simulink model "downlink_4c2t"  (Simulink 8.7)
settings: Solver=VariableStepDiscrete  StartTime=0.0  StopTime=DUC_LINEUP_param.endTime  RelTol=1e-3
PreLoadFcn:
  | % Run the setup script when the model is opened
  | setup_downlink_4c2t;
InitFcn:
  | % Run the setup script again just before the
  | % model is run, so that any updates made
  | % after opening are applied.
  | setup_downlink_4c2t;
  | 
  | %% DSPBuilder Start
  | alt_dspbuilder_update_model(bdroot)
  | %% DSPBuilder End
values from neighbouring files (symbols this model uses):
  LUTS_DPD_CLIP =     [downlink_4c2t_dpd_clip.mat]
  PulsExtention = 128    [setup_downlink_4c2t.m]
  StartAddress1 = Iter1_Param.BaseAddr + 3200    [setup_downlink_4c2t.m]
  StartAddress2 = StartAddress1+1024    [setup_downlink_4c2t.m]
  win = [w(1:PulsExtention) ones(1,Iter0_Param.pulseLen) w(PulsExtention+1:end)]    [setup_downlink_4c2t.m]
undefined symbols (not defined in the file or in its folder): AdvDSPBChannelOutDisplay, AdvDSPBDMemDisplay, dpoly, dspba_ChannelInVis, dspba_ChannelOutVis, dspba_internal_get_channel_ports, dspba_internal_get_demux_ports, DUC_LINEUP_param, evalAionMaskParam, iq_width, Iter0_Param, latency, primtype, REG, UseDontCare, value
undefined symbols (not defined in the file): cfr0_id, cfr_Params0, cfr_Params1, clock_rate, REG_dut_id_addr
libraries: DSPBAPrim x1438, DSPBAControl x77, DSPBAModelBus x71, DSPBABase x40, downlink_4c2t_foldingcfr_3firs_lib x26, DSPBAUtilities x8, downlink_4c2t_lib x4, downlink_4c2t_cordic_lib x2, downlink_4c2t_dpd_clipper x2, DSPBAFilters x2, DSPBAWaveformSynth x2, downlink_4c2t_lduc_lib x1
(part 13 of 17)

== system downlink_4c2t/DUT/DUC_IN_PM/carrier_separation/Subsystem4 ==
  channel_in : Inport
  valid_in : Inport  Port=2
  axc0_dataout : Inport  Port=3
  axc1_dataout : Inport  Port=4
  axc2_dataout : Inport  Port=5
  axc3_dataout : Inport  Port=6
  axc4_dataout : Inport  Port=7
  axc5_dataout : Inport  Port=8
  axc6_dataout : Inport  Port=9
  axc7_dataout : Inport  Port=10
  BitExtract1 : DSPBAPrim/BitExtract  primtype=bitextract  nInputs=1  nOutputs=1  omode=Specify via dialog  otype=ufix(4)  scale=2^0  rndmethod=Unbiased  factor=1  satmethod=Symmetric  shift_vec=[0 1 2 -1]  value=1  inPortNames=[' '; ' ';]  outPortNames=[' ']  dspbaimage=dspba_prim.jpg  text=fprintf('..%d', value);  style=Optimised  visibilities=8 + 1024  version=20090407
  Const : DSPBAPrim/Const  primtype=const  nInputs=0  nOutputs=1  omode=Inherit via internal rule  otype=sfix(16)  scale=2^-15  rndmethod=Unbiased  factor=1  satmethod=Symmetric  shift_vec=[0 1 2 -1]  value=0  inPortNames=['+'; '+';]  outPortNames=[' ']  dspbaimage=dspba_prim.jpg  text=fprintf('%s', num2str(value));  style=Optimised  visibilities=8 + 1024  floatPrecision=float32_m23  version=20120820
  Const1 : DSPBAPrim/Const  primtype=const  nInputs=0  nOutputs=1  omode=Inherit via internal rule  otype=sfix(16)  scale=2^-15  rndmethod=Unbiased  factor=1  satmethod=Symmetric  shift_vec=[0 1 2 -1]  value=1  inPortNames=['+'; '+';]  outPortNames=[' ']  dspbaimage=dspba_prim.jpg  text=fprintf('%s', num2str(value));  style=Optimised  visibilities=8 + 1024  floatPrecision=float32_m23  version=20120820
  Const2 : DSPBAPrim/Const  primtype=const  nInputs=0  nOutputs=1  omode=Inherit via internal rule  otype=sfix(16)  scale=2^-15  rndmethod=Unbiased  factor=1  satmethod=Symmetric  shift_vec=[0 1 2 -1]  value=2  inPortNames=['+'; '+';]  outPortNames=[' ']  dspbaimage=dspba_prim.jpg  text=fprintf('%s', num2str(value));  style=Optimised  visibilities=8 + 1024  floatPrecision=float32_m23  version=20120820
  Const3 : DSPBAPrim/Const  primtype=const  nInputs=0  nOutputs=1  omode=Inherit via internal rule  otype=sfix(16)  scale=2^-15  rndmethod=Unbiased  factor=1  satmethod=Symmetric  shift_vec=[0 1 2 -1]  value=3  inPortNames=['+'; '+';]  outPortNames=[' ']  dspbaimage=dspba_prim.jpg  text=fprintf('%s', num2str(value));  style=Optimised  visibilities=8 + 1024  floatPrecision=float32_m23  version=20120820
  Const4 : DSPBAPrim/Const  primtype=const  nInputs=0  nOutputs=1  omode=Inherit via internal rule  otype=sfix(16)  scale=2^-15  rndmethod=Unbiased  factor=1  satmethod=Symmetric  shift_vec=[0 1 2 -1]  value=4  inPortNames=['+'; '+';]  outPortNames=[' ']  dspbaimage=dspba_prim.jpg  text=fprintf('%s', num2str(value));  style=Optimised  visibilities=8 + 1024  floatPrecision=float32_m23  version=20120820
  Const5 : DSPBAPrim/Const  primtype=const  nInputs=0  nOutputs=1  omode=Inherit via internal rule  otype=sfix(16)  scale=2^-15  rndmethod=Unbiased  factor=1  satmethod=Symmetric  shift_vec=[0 1 2 -1]  value=5  inPortNames=['+'; '+';]  outPortNames=[' ']  dspbaimage=dspba_prim.jpg  text=fprintf('%s', num2str(value));  style=Optimised  visibilities=8 + 1024  floatPrecision=float32_m23  version=20120820
  Const6 : DSPBAPrim/Const  primtype=const  nInputs=0  nOutputs=1  omode=Inherit via internal rule  otype=sfix(16)  scale=2^-15  rndmethod=Unbiased  factor=1  satmethod=Symmetric  shift_vec=[0 1 2 -1]  value=6  inPortNames=['+'; '+';]  outPortNames=[' ']  dspbaimage=dspba_prim.jpg  text=fprintf('%s', num2str(value));  style=Optimised  visibilities=8 + 1024  floatPrecision=float32_m23  version=20120820
  Const7 : DSPBAPrim/Const  primtype=const  nInputs=0  nOutputs=1  omode=Inherit via internal rule  otype=sfix(16)  scale=2^-15  rndmethod=Unbiased  factor=1  satmethod=Symmetric  shift_vec=[0 1 2 -1]  value=7  inPortNames=['+'; '+';]  outPortNames=[' ']  dspbaimage=dspba_prim.jpg  text=fprintf('%s', num2str(value));  style=Optimised  visibilities=8 + 1024  floatPrecision=float32_m23  version=20120820
  Subsystem : Subsystem
  Subsystem1 : Subsystem
  Subsystem10 : Subsystem
  Subsystem11 : Subsystem
  Subsystem12 : Subsystem
  Subsystem13 : Subsystem
  Subsystem14 : Subsystem
  Subsystem15 : Subsystem
  Subsystem2 : Subsystem
  Subsystem3 : Subsystem
  Subsystem4 : Subsystem
  Subsystem5 : Subsystem
  Subsystem6 : Subsystem
  Subsystem7 : Subsystem
  Subsystem8 : Subsystem
  Subsystem9 : Subsystem
  axc0_valid_out : Outport
  "axc0_data_out " : Outport  Port=2
  axc1_valid_out : Outport  Port=3
  axc1_data_out : Outport  Port=4
  axc2_valid_out : Outport  Port=5
  axc2_data_out : Outport  Port=6
  axc3_valid_out : Outport  Port=7
  axc3_data_out : Outport  Port=8
  axc4_valid_out : Outport  Port=9
  axc4_data_out : Outport  Port=10
  axc5_valid_out : Outport  Port=11
  axc5_data_out : Outport  Port=12
  axc6_valid_out : Outport  Port=13
  axc6_data_out : Outport  Port=14
  axc7_valid_out : Outport  Port=15
  axc7_data_out : Outport  Port=16
  wires:
  Const1/1 -> Subsystem1/2(channel_num)
  Const3/1 -> Subsystem3/2(channel_num)
  Const2/1 -> Subsystem2/2(channel_num)
  Const/1 -> Subsystem/2(channel_num)
  Subsystem/1(valid_out) -> Subsystem4/1(valid_in)
  Subsystem1/1(valid_out) -> Subsystem5/1(valid_in)
  Subsystem2/1(valid_out) -> Subsystem6/1(valid_in)
  Subsystem3/1(valid_out) -> Subsystem7/1(valid_in)
  axc0_dataout/1 -> Subsystem4/2("data_in ")
  axc1_dataout/1 -> Subsystem5/2("data_in ")
  axc2_dataout/1 -> Subsystem6/2("data_in ")
  axc3_dataout/1 -> Subsystem7/2("data_in ")
  Const4/1 -> Subsystem8/2(channel_num)
  Subsystem8/1(valid_out) -> Subsystem9/1(valid_in)
  axc4_dataout/1 -> Subsystem9/2("data_in ")
  Const6/1 -> Subsystem11/2(channel_num)
  Const5/1 -> Subsystem10/2(channel_num)
  Subsystem10/1(valid_out) -> Subsystem12/1(valid_in)
  Subsystem11/1(valid_out) -> Subsystem13/1(valid_in)
  axc5_dataout/1 -> Subsystem12/2("data_in ")
  axc6_dataout/1 -> Subsystem13/2("data_in ")
  Const7/1 -> Subsystem14/2(channel_num)
  valid_in/1 -> Subsystem10/3(valid_in), Subsystem11/3(valid_in), Subsystem14/3(valid_in), Subsystem8/3(valid_in), Subsystem3/3(valid_in), Subsystem2/3(valid_in), Subsystem1/3(valid_in), Subsystem/3(valid_in)
  channel_in/1 -> BitExtract1/1
  Subsystem14/1(valid_out) -> Subsystem15/1(valid_in)
  axc7_dataout/1 -> Subsystem15/2("data_in ")
  Subsystem4/2("data_out ") -> "axc0_data_out "/1
  Subsystem7/1(vaid_out) -> axc3_valid_out/1
  Subsystem4/1(vaid_out) -> axc0_valid_out/1
  Subsystem5/1(vaid_out) -> axc1_valid_out/1
  Subsystem5/2("data_out ") -> axc1_data_out/1
  Subsystem6/1(vaid_out) -> axc2_valid_out/1
  Subsystem6/2("data_out ") -> axc2_data_out/1
  Subsystem12/2("data_out ") -> axc5_data_out/1
  Subsystem13/1(vaid_out) -> axc6_valid_out/1
  Subsystem13/2("data_out ") -> axc6_data_out/1
  Subsystem15/1(vaid_out) -> axc7_valid_out/1
  Subsystem15/2("data_out ") -> axc7_data_out/1
  Subsystem7/2("data_out ") -> axc3_data_out/1
  Subsystem12/1(vaid_out) -> axc5_valid_out/1
  Subsystem9/2("data_out ") -> axc4_data_out/1
  Subsystem9/1(vaid_out) -> axc4_valid_out/1
  BitExtract1/1 -> Subsystem1/1(channel_in), Subsystem10/1(channel_in), Subsystem11/1(channel_in), Subsystem14/1(channel_in), Subsystem8/1(channel_in), Subsystem3/1(channel_in), Subsystem2/1(channel_in), Subsystem/1(channel_in)

== system downlink_4c2t/DUT/DUC_SUMMER_PM/Ant1_accumulator/neg_egde ==
  In1 : Inport
  And : DSPBAPrim/And  primtype=and  nInputs=2  nOutputs=1  omode=Inherit via internal rule  otype=sfix(16)  scale=2^-15  rndmethod=Unbiased  factor=1  satmethod=Symmetric  shift_vec=[0 1 2 -1]  value=0  inPortNames=[' '; ' '; ' '; ' '; ' '; ' '; ' '; ' '; ' '; ' '; ' '; ' '; ' '; ' '; ' '; ' '; ]  outPortNames=[' ']  dspbaimage=dspba_prim.jpg  text=fprintf('&');  style=Optimised  visibilities=8+2  version=20090407
  Not : DSPBAPrim/Not  primtype=not  nInputs=1  nOutputs=1  omode=Inherit via internal rule  otype=sfix(16)  scale=2^-15  rndmethod=Unbiased  factor=1  satmethod=Symmetric  shift_vec=[0 1 2 -1]  value=0  inPortNames=[' '; ' ';]  outPortNames=[' ']  dspbaimage=dspba_prim.jpg  text=fprintf('~');  style=Optimised  visibilities=8  version=20090407
  SampleDelay3 : DSPBAPrim/SampleDelay  primtype=sampdelay  nInputs=1  nOutputs=1  omode=Inherit via internal rule  otype=sfix(16)  scale=2^-15  rndmethod=Unbiased  factor=1  satmethod=Symmetric  shift_vec=[0 1 2 -1]  value=1  inPortNames=[' '; ' ';]  outPortNames=[' ']  dspbaimage=dspba_prim.jpg  text=dpoly(1, eye(1,value+1), 'z')  style=Optimised  visibilities=8 + 1024 + 2^17 + 2^18  flexible=off  slackgroup=0  augmented=0  version=20090407  advOptions=[]
  Out1 : Outport
  wires:
  In1/1 -> Not/1, SampleDelay3/1
  SampleDelay3/1 -> And/1
  Not/1 -> And/2
  And/1 -> Out1/1

== system downlink_4c2t/DUT/DUC_SUMMER_PM/Ant2_accumulator/neg_egde ==
  In1 : Inport
  And : DSPBAPrim/And  primtype=and  nInputs=2  nOutputs=1  omode=Inherit via internal rule  otype=sfix(16)  scale=2^-15  rndmethod=Unbiased  factor=1  satmethod=Symmetric  shift_vec=[0 1 2 -1]  value=0  inPortNames=[' '; ' '; ' '; ' '; ' '; ' '; ' '; ' '; ' '; ' '; ' '; ' '; ' '; ' '; ' '; ' '; ]  outPortNames=[' ']  dspbaimage=dspba_prim.jpg  text=fprintf('&');  style=Optimised  visibilities=8+2  version=20090407
  Not : DSPBAPrim/Not  primtype=not  nInputs=1  nOutputs=1  omode=Inherit via internal rule  otype=sfix(16)  scale=2^-15  rndmethod=Unbiased  factor=1  satmethod=Symmetric  shift_vec=[0 1 2 -1]  value=0  inPortNames=[' '; ' ';]  outPortNames=[' ']  dspbaimage=dspba_prim.jpg  text=fprintf('~');  style=Optimised  visibilities=8  version=20090407
  SampleDelay3 : DSPBAPrim/SampleDelay  primtype=sampdelay  nInputs=1  nOutputs=1  omode=Inherit via internal rule  otype=sfix(16)  scale=2^-15  rndmethod=Unbiased  factor=1  satmethod=Symmetric  shift_vec=[0 1 2 -1]  value=1  inPortNames=[' '; ' ';]  outPortNames=[' ']  dspbaimage=dspba_prim.jpg  text=dpoly(1, eye(1,value+1), 'z')  style=Optimised  visibilities=8 + 1024 + 2^17 + 2^18  flexible=off  slackgroup=0  augmented=0  version=20090407  advOptions=[]
  Out1 : Outport
  wires:
  In1/1 -> Not/1, SampleDelay3/1
  SampleDelay3/1 -> And/1
  Not/1 -> And/2
  And/1 -> Out1/1

== system downlink_4c2t/DUT/DUC_SUMMER_PM/carrier_separation/Subsystem4 ==
  channel_in : Inport
  valid_in : Inport  Port=2
  axc0_dataout : Inport  Port=3
  axc1_dataout : Inport  Port=4
  BitExtract1 : DSPBAPrim/BitExtract  primtype=bitextract  nInputs=1  nOutputs=1  omode=Specify via dialog  otype=ufix(2)  scale=2^0  rndmethod=Unbiased  factor=1  satmethod=Symmetric  shift_vec=[0 1 2 -1]  value=1  inPortNames=[' '; ' ';]  outPortNames=[' ']  dspbaimage=dspba_prim.jpg  text=fprintf('..%d', value);  style=Optimised  visibilities=8 + 1024  version=20090407
  Const : DSPBAPrim/Const  primtype=const  nInputs=0  nOutputs=1  omode=Inherit via internal rule  otype=sfix(16)  scale=2^-15  rndmethod=Unbiased  factor=1  satmethod=Symmetric  shift_vec=[0 1 2 -1]  value=0  inPortNames=['+'; '+';]  outPortNames=[' ']  dspbaimage=dspba_prim.jpg  text=fprintf('%s', num2str(value));  style=Optimised  visibilities=8 + 1024  floatPrecision=float32_m23  version=20120820
  Const1 : DSPBAPrim/Const  primtype=const  nInputs=0  nOutputs=1  omode=Inherit via internal rule  otype=sfix(16)  scale=2^-15  rndmethod=Unbiased  factor=1  satmethod=Symmetric  shift_vec=[0 1 2 -1]  value=1  inPortNames=['+'; '+';]  outPortNames=[' ']  dspbaimage=dspba_prim.jpg  text=fprintf('%s', num2str(value));  style=Optimised  visibilities=8 + 1024  floatPrecision=float32_m23  version=20120820
  Subsystem : Subsystem
  Subsystem1 : Subsystem
  Subsystem2 : Subsystem
  Subsystem4 : Subsystem
  axc0_valid_out : Outport
  "axc0_data_out " : Outport  Port=2
  axc1_valid_out : Outport  Port=3
  axc1_data_out : Outport  Port=4
  wires:
  BitExtract1/1 -> Subsystem/1(channel_in), Subsystem1/1(channel_in)
  Subsystem2/2("data_out ") -> axc1_data_out/1
  Subsystem2/1(vaid_out) -> axc1_valid_out/1
  Subsystem4/1(vaid_out) -> axc0_valid_out/1
  Subsystem4/2("data_out ") -> "axc0_data_out "/1
  channel_in/1 -> BitExtract1/1
  valid_in/1 -> Subsystem/3(valid_in), Subsystem1/3(valid_in)
  axc1_dataout/1 -> Subsystem2/2("data_in ")
  axc0_dataout/1 -> Subsystem4/2("data_in ")
  Subsystem1/1(valid_out) -> Subsystem2/1(valid_in)
  Subsystem/1(valid_out) -> Subsystem4/1(valid_in)
  Const/1 -> Subsystem/2(channel_num)
  Const1/1 -> Subsystem1/2(channel_num)

== system downlink_4c2t/DUT/LDUC/Mixer_Summer/COMPLEX_MIXER ==
  a : Inport
  v : Inport  Port=2
  c : Inport  Port=3
  sync_pulse : Inport  Port=4
  ComplexMixer : DSPBAWaveformSynth/ComplexMixer  nInputRate=DUC_LINEUP_param.CM.SampleRate  nchan=DUC_LINEUP_param.CM.No_Of_Complex_chan  nfreq=DUC_LINEUP_param.CM.No_Of_Complex_Freq  latency=4  version=20090407
  Const1 : DSPBAPrim/Const  primtype=const  nInputs=0  nOutputs=1  omode=Specify via dialog  otype=ufix(24)  scale=2^-0  rndmethod=Unbiased  factor=1  satmethod=Symmetric  shift_vec=[0 1 2 -1]  value=[0 0]  inPortNames=['+'; '+';]  outPortNames=[' ']  dspbaimage=dspba_prim.jpg  text=fprintf('%s', num2str(value));  style=Optimised  visibilities=8 + 1024  floatPrecision=float32_m23  version=20120820
  Const25 : DSPBAPrim/Const  primtype=const  nInputs=0  nOutputs=1  omode=Inherit via internal rule  otype=sfix(16)  scale=2^-15  rndmethod=Unbiased  factor=1  satmethod=Symmetric  shift_vec=[0 1 2 -1]  value=0  inPortNames=['+'; '+';]  outPortNames=[' ']  dspbaimage=dspba_prim.jpg  text=fprintf('%s', num2str(value));  style=Optimised  visibilities=8 + 1024  floatPrecision=float32_m23  version=20120820
  Delay Module : Subsystem
  Demux : Demux  Outputs=2
  IQ_Splitter : Subsystem
  Mux : Mux  Inputs=2
  Mux1 : Mux  Inputs=2
  NCO1 : DSPBAWaveformSynth/NCO  outputRate=DUC_LINEUP_param.NCO.SampleRate  otype=sfix(DUC_LINEUP_param.NCO.Data_type)  scale=2^-DUC_LINEUP_param.NCO.scaling_value  expSFDR=96.32  accumBitWidth=DUC_LINEUP_param.NCO.Acumulater_bit_wid  accumPrecision=+/- 3.6621  phaseIncrAndInv=DUC_LINEUP_param.A12xC_NCO.Freq_word  phaseIncrInMHz="[0  0  0  0  0  0  0  0]"  phaseIncrAndInvMap=DUC_LINEUP_param.A12xC_NCO.base_addr  rwmode=Read/Write  exposebus=off  outWidth=2  tableSize=8  latency=19  version=20090407
  Terminator28 : Terminator
  Terminator8 : Terminator
  Terminator9 : Terminator
  scale1_ComplexMixer : DSPBABase/Scale  otype=sfix(DUC_LINEUP_param.output_word_length)  scale=2^-DUC_LINEUP_param.output_fraction_length  rndmethod=Truncate  factor=[1 1]  satmethod=Symmetric  shift_vec=[0 0]  latency=6  wideSimulation=off  version=20090407
  out_I : Outport
  out_q : Outport  Port=2
  q_v : Outport  Port=3
  q_c : Outport  Port=4
  wires:
  Delay Module/4(Out_Chan) -> Terminator9/1
  v/1 -> IQ_Splitter/2(valid)
  NCO1/1 -> ComplexMixer/5
  Delay Module/3(Out_Valid) -> Terminator8/1
  ComplexMixer/1 -> Mux/1
  scale1_ComplexMixer/3 -> q_c/1
  scale1_ComplexMixer/4 -> Terminator28/1
  Mux/1 -> scale1_ComplexMixer/1
  IQ_Splitter/4(Out_channel) -> Delay Module/4(In_Chann), NCO1/1
  scale1_ComplexMixer/2 -> q_v/1
  c/1 -> IQ_Splitter/3(channel)
  ComplexMixer/2 -> Mux/2
  IQ_Splitter/1(Out_data_I) -> Delay Module/1(In_Data1)
  ComplexMixer/3 -> scale1_ComplexMixer/2
  a/1 -> IQ_Splitter/1(data)
  Delay Module/1(Out_Data1) -> ComplexMixer/1
  NCO1/3 -> ComplexMixer/3
  ComplexMixer/4 -> scale1_ComplexMixer/3
  NCO1/4 -> ComplexMixer/4
  NCO1/2 -> ComplexMixer/6
  Const1/1 -> NCO1/3
  Const25/1 -> scale1_ComplexMixer/4
  scale1_ComplexMixer/1 -> Demux/1
  Demux/1 -> out_I/1
  Demux/2 -> out_q/1
  IQ_Splitter/2(Out_data_Q) -> Delay Module/2(In_Data2)
  IQ_Splitter/3(Out_valid) -> NCO1/2, Delay Module/3(In_Valid)
  Mux1/1 -> NCO1/4
  sync_pulse/1 -> Mux1/2, Mux1/1
  Delay Module/2(Out_Data2) -> ComplexMixer/2

== system downlink_4c2t/DUT/LDUC/Mixer_Summer/SUMMER ==
  a : Inport
  a1 : Inport  Port=2
  v : Inport  Port=3
  c : Inport  Port=4
  sum_shift : Inport  Port=5
  IQ_Summer : Subsystem
  Terminator7 : Terminator
  scale_HB_filter5 : DSPBABase/Scale  otype=sfix(DUC_LINEUP_param.output_word_length)  scale=2^-DUC_LINEUP_param.output_fraction_length  rndmethod=Truncate  factor=1  satmethod=Symmetric  shift_vec=[0 -1 -2 -2]  latency=6  wideSimulation=off  version=20090407
  q : Outport
  q_v : Outport  Port=2
  q_c : Outport  Port=3
  wires:
  v/1 -> IQ_Summer/3(valid)
  c/1 -> IQ_Summer/4(chann)
  scale_HB_filter5/2 -> q_v/1
  scale_HB_filter5/3 -> q_c/1
  scale_HB_filter5/4 -> Terminator7/1
  IQ_Summer/2(out_valid) -> scale_HB_filter5/2
  a/1 -> IQ_Summer/1(data0)
  scale_HB_filter5/1 -> q/1
  IQ_Summer/1(Out_data) -> scale_HB_filter5/1
  IQ_Summer/3(Out_chann) -> scale_HB_filter5/3
  a1/1 -> IQ_Summer/2(data1)
  sum_shift/1 -> scale_HB_filter5/4

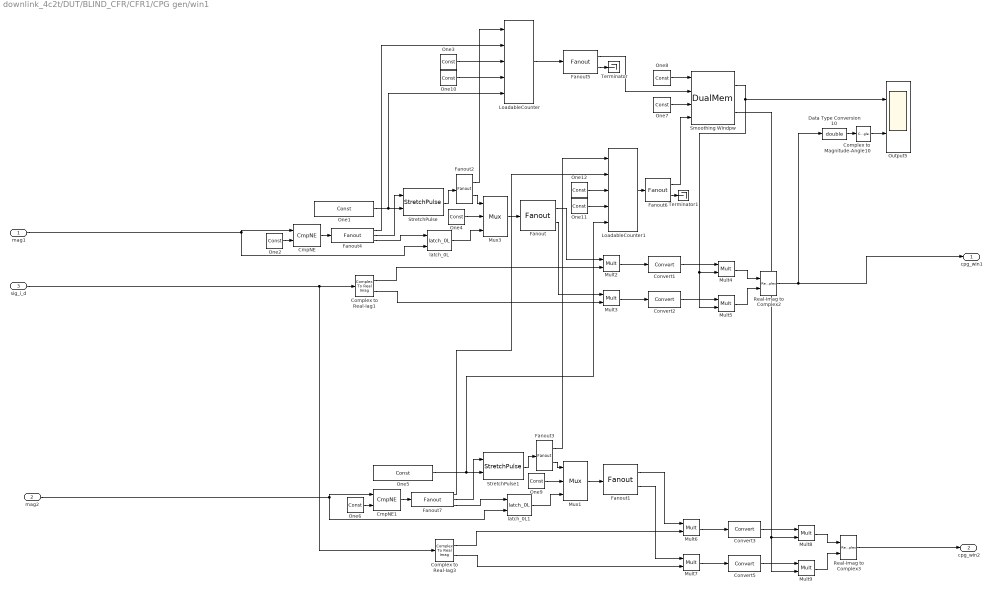
== system downlink_4c2t/DUT/BLIND_CFR/CFR1/CPG gen/win1 ==
  mag1 : Inport
  mag2 : Inport  Port=2
  sig_i_d : Inport  Port=3
  CmpNE : DSPBAPrim/CmpNE  primtype=cmpne  nInputs=2  nOutputs=1  omode=boolean  otype=sfix(16)  scale=2^-15  rndmethod=Unbiased  factor=1  satmethod=Symmetric  shift_vec=[0 1 2 -1]  value=0  inPortNames=[' '; ' ';]  outPortNames=[' ']  dspbaimage=dspba_prim.jpg  text=fprintf('~=');  style=Optimised  visibilities=0  advOptions=[]  version=20130117
  CmpNE1 : DSPBAPrim/CmpNE  primtype=cmpne  nInputs=2  nOutputs=1  omode=boolean  otype=sfix(16)  scale=2^-15  rndmethod=Unbiased  factor=1  satmethod=Symmetric  shift_vec=[0 1 2 -1]  value=0  inPortNames=[' '; ' ';]  outPortNames=[' ']  dspbaimage=dspba_prim.jpg  text=fprintf('~=');  style=Optimised  visibilities=0  advOptions=[]  version=20130117
  Complex to Magnitude-Angle10 : ComplexToMagnitudeAngle  Output=Magnitude
  Complex to Real-Iag1 : ComplexToRealImag
  Complex to Real-Iag3 : ComplexToRealImag
  Convert{1..3,5} (4 alike) : DSPBAPrim/Convert  primtype=convert  nInputs=1  nOutputs=1  omode=Specify via dialog  otype=sfix(16)  scale=2^-(15)  rndmethod=Unbiased  factor=1  satmethod=None  shift_vec=[0 1 2 -1]  value=round([0:255]/17)  inPortNames=[' '; ' ';]  outPortNames=[' '; 'c']  dspbaimage=dspba_prim.jpg  text=fprintf('convert');  style=Optimised  visibilities=8+64+256  clipdetect=off  floatPrecision=float32_m23  advOptions=[]  version=20130211
  Data Type Conversion10 : DataTypeConversion  OutDataTypeStr=double
  Fanout{,1..3,5..6} (6 alike) : DSPBAPrim/Fanout  primtype=fanout  nInputs=1  nOutputs=evalAionMaskParam(gcb,'value',1)  omode=Inherit via internal rule  otype=sfix(16)  scale=2^-15  rndmethod=Unbiased  factor=1  satmethod=Symmetric  shift_vec=[0 1 2 -1]  value=2  inPortNames=[' '; ' ';]  outPortNames=[' ']  dspbaimage=dspba_prim.jpg  text=fprintf('fanout')  style=Optimised  visibilities=2^10+2^18  version=20150501  uninit=off
  Fanout4 : DSPBAPrim/Fanout  primtype=fanout  nInputs=1  nOutputs=evalAionMaskParam(gcb,'value',1)  omode=Inherit via internal rule  otype=sfix(16)  scale=2^-15  rndmethod=Unbiased  factor=1  satmethod=Symmetric  shift_vec=[0 1 2 -1]  value=3  inPortNames=[' '; ' ';]  outPortNames=[' ']  dspbaimage=dspba_prim.jpg  text=fprintf('fanout')  style=Optimised  visibilities=2^10+2^18  version=20150501  uninit=off
  Fanout7 : DSPBAPrim/Fanout  primtype=fanout  nInputs=1  nOutputs=evalAionMaskParam(gcb,'value',1)  omode=Inherit via internal rule  otype=sfix(16)  scale=2^-15  rndmethod=Unbiased  factor=1  satmethod=Symmetric  shift_vec=[0 1 2 -1]  value=3  inPortNames=[' '; ' ';]  outPortNames=[' ']  dspbaimage=dspba_prim.jpg  text=fprintf('fanout')  style=Optimised  visibilities=2^10+2^18  version=20150501  uninit=off
  LoadableCounter : DSPBAPrim/LoadableCounter  primtype=loadablecounter  nInputs=5  nOutputs=1  omode=Inherit via internal rule  otype=ufix(16)  scale=2^-0  rndmethod=Unbiased  factor=1  satmethod=Symmetric  shift_vec=[0 1 2 -1]  value=[0 length(win) 1]  inPortNames=['en';'ld';'i ';'s ';'m ']  outPortNames=[' ']  dspbaimage=dspba_prim.jpg  text=fprintf('loadable\ncounter\n[%d %d %d]', value(1), value(2), value(3));  style=Optimised  visibilities=8 + 1024  version=20090407
  LoadableCounter1 : DSPBAPrim/LoadableCounter  primtype=loadablecounter  nInputs=5  nOutputs=1  omode=Inherit via internal rule  otype=ufix(16)  scale=2^-0  rndmethod=Unbiased  factor=1  satmethod=Symmetric  shift_vec=[0 1 2 -1]  value=[0 length(win) 1]  inPortNames=['en';'ld';'i ';'s ';'m ']  outPortNames=[' ']  dspbaimage=dspba_prim.jpg  text=fprintf('loadable\ncounter\n[%d %d %d]', value(1), value(2), value(3));  style=Optimised  visibilities=8 + 1024  version=20090407
  Mult{2..9} (8 alike) : DSPBAPrim/Mult  primtype=mult  nInputs=2  nOutputs=1  omode=Inherit via internal rule  otype=sfix(16)  scale=2^-15  rndmethod=Unbiased  factor=1  satmethod=Symmetric  shift_vec=[0 1 2 -1]  value=0  inPortNames=[' '; ' ';]  outPortNames=[' ']  dspbaimage=dspba_prim.jpg  text=fprintf('X');  style=Optimised  visibilities=8+2^18+2^19  floatPrecision=float32_m23  floatRounding=correct  advOptions=[]  version=20130115
  Mux1 : DSPBAPrim/Mux  primtype=mux  nInputs=evalAionMaskParam(gcb,'value',1)+1  nOutputs=1  omode=Inherit via internal rule  otype=sfix(16)  scale=2^-15  rndmethod=Unbiased  factor=1  satmethod=Symmetric  shift_vec=[0 1 2 -1]  value=2  inPortNames=['s'; 'd0'; 'd1'; 'd2'; 'd3'; 'd4'; 'd5'; 'd6'; 'd7'; 'd8'; 'd9';]  outPortNames=[' ']  dspbaimage=dspba_prim.jpg  text=fprintf('%s', primtype);  style=Optimised  visibilities=1032  version=20131025
  Mux3 : DSPBAPrim/Mux  primtype=mux  nInputs=evalAionMaskParam(gcb,'value',1)+1  nOutputs=1  omode=Inherit via internal rule  otype=sfix(16)  scale=2^-15  rndmethod=Unbiased  factor=1  satmethod=Symmetric  shift_vec=[0 1 2 -1]  value=2  inPortNames=['s'; 'd0'; 'd1'; 'd2'; 'd3'; 'd4'; 'd5'; 'd6'; 'd7'; 'd8'; 'd9';]  outPortNames=[' ']  dspbaimage=dspba_prim.jpg  text=fprintf('%s', primtype);  style=Optimised  visibilities=1032  version=20131025
  One1 : DSPBAPrim/Const  primtype=const  nInputs=0  nOutputs=1  omode=Specify via dialog  otype=uint(10)  scale=2^0  rndmethod=Unbiased  factor=1  satmethod=Symmetric  shift_vec=[0 1 2 -1]  value=Iter0_Param.winLen  inPortNames=['+'; '+';]  outPortNames=[' ']  dspbaimage=dspba_prim.jpg  text=fprintf('%s', num2str(value));  style=Optimised  visibilities=8 + 1024  floatPrecision=float32_m23  version=20120820
  One10 : DSPBAPrim/Const  primtype=const  nInputs=0  nOutputs=1  omode=Specify via dialog  otype=uint(10)  scale=2^0  rndmethod=Unbiased  factor=1  satmethod=Symmetric  shift_vec=[0 1 2 -1]  value=1  inPortNames=['+'; '+';]  outPortNames=[' ']  dspbaimage=dspba_prim.jpg  text=fprintf('%s', num2str(value));  style=Optimised  visibilities=8 + 1024  floatPrecision=float32_m23  version=20120820
  One11 : DSPBAPrim/Const  primtype=const  nInputs=0  nOutputs=1  omode=Specify via dialog  otype=uint(10)  scale=2^0  rndmethod=Unbiased  factor=1  satmethod=Symmetric  shift_vec=[0 1 2 -1]  value=1  inPortNames=['+'; '+';]  outPortNames=[' ']  dspbaimage=dspba_prim.jpg  text=fprintf('%s', num2str(value));  style=Optimised  visibilities=8 + 1024  floatPrecision=float32_m23  version=20120820
  One12 : DSPBAPrim/Const  primtype=const  nInputs=0  nOutputs=1  omode=Specify via dialog  otype=uint(10)  scale=2^0  rndmethod=Unbiased  factor=1  satmethod=Symmetric  shift_vec=[0 1 2 -1]  value=0  inPortNames=['+'; '+';]  outPortNames=[' ']  dspbaimage=dspba_prim.jpg  text=fprintf('%s', num2str(value));  style=Optimised  visibilities=8 + 1024  floatPrecision=float32_m23  version=20120820
  One2 : DSPBAPrim/Const  primtype=const  nInputs=0  nOutputs=1  omode=Inherit via internal rule  otype=sfix(16)  scale=2^-15  rndmethod=Unbiased  factor=1  satmethod=Symmetric  shift_vec=[0 1 2 -1]  value=0  inPortNames=['+'; '+';]  outPortNames=[' ']  dspbaimage=dspba_prim.jpg  text=fprintf('%s', num2str(value));  style=Optimised  visibilities=8 + 1024  floatPrecision=float32_m23  version=20120820
  One3 : DSPBAPrim/Const  primtype=const  nInputs=0  nOutputs=1  omode=Specify via dialog  otype=uint(10)  scale=2^0  rndmethod=Unbiased  factor=1  satmethod=Symmetric  shift_vec=[0 1 2 -1]  value=0  inPortNames=['+'; '+';]  outPortNames=[' ']  dspbaimage=dspba_prim.jpg  text=fprintf('%s', num2str(value));  style=Optimised  visibilities=8 + 1024  floatPrecision=float32_m23  version=20120820
  One4 : DSPBAPrim/Const  primtype=const  nInputs=0  nOutputs=1  omode=Specify via dialog  otype=ufix(16)  scale=2^-15  rndmethod=Unbiased  factor=1  satmethod=Symmetric  shift_vec=[0 1 2 -1]  value=0  inPortNames=['+'; '+';]  outPortNames=[' ']  dspbaimage=dspba_prim.jpg  text=fprintf('%s', num2str(value));  style=Optimised  visibilities=8 + 1024  floatPrecision=float32_m23  version=20120820
  One5 : DSPBAPrim/Const  primtype=const  nInputs=0  nOutputs=1  omode=Specify via dialog  otype=uint(10)  scale=2^0  rndmethod=Unbiased  factor=1  satmethod=Symmetric  shift_vec=[0 1 2 -1]  value=Iter0_Param.winLen  inPortNames=['+'; '+';]  outPortNames=[' ']  dspbaimage=dspba_prim.jpg  text=fprintf('%s', num2str(value));  style=Optimised  visibilities=8 + 1024  floatPrecision=float32_m23  version=20120820
  One6 : DSPBAPrim/Const  primtype=const  nInputs=0  nOutputs=1  omode=Inherit via internal rule  otype=sfix(16)  scale=2^-15  rndmethod=Unbiased  factor=1  satmethod=Symmetric  shift_vec=[0 1 2 -1]  value=0  inPortNames=['+'; '+';]  outPortNames=[' ']  dspbaimage=dspba_prim.jpg  text=fprintf('%s', num2str(value));  style=Optimised  visibilities=8 + 1024  floatPrecision=float32_m23  version=20120820
  One7 : DSPBAPrim/Const  primtype=const  nInputs=0  nOutputs=1  omode=boolean  otype=sfix(16)  scale=2^-15  rndmethod=Unbiased  factor=1  satmethod=Symmetric  shift_vec=[0 1 2 -1]  value=0  inPortNames=['+'; '+';]  outPortNames=[' ']  dspbaimage=dspba_prim.jpg  text=fprintf('%s', num2str(value));  style=Optimised  visibilities=8 + 1024  floatPrecision=float32_m23  version=20120820
  One8 : DSPBAPrim/Const  primtype=const  nInputs=0  nOutputs=1  omode=Specify via dialog  otype=sfix(16)  scale=2^-15  rndmethod=Unbiased  factor=1  satmethod=Symmetric  shift_vec=[0 1 2 -1]  value=0  inPortNames=['+'; '+';]  outPortNames=[' ']  dspbaimage=dspba_prim.jpg  text=fprintf('%s', num2str(value));  style=Optimised  visibilities=8 + 1024  floatPrecision=float32_m23  version=20120820
  One9 : DSPBAPrim/Const  primtype=const  nInputs=0  nOutputs=1  omode=Specify via dialog  otype=ufix(16)  scale=2^-15  rndmethod=Unbiased  factor=1  satmethod=Symmetric  shift_vec=[0 1 2 -1]  value=0  inPortNames=['+'; '+';]  outPortNames=[' ']  dspbaimage=dspba_prim.jpg  text=fprintf('%s', num2str(value));  style=Optimised  visibilities=8 + 1024  floatPrecision=float32_m23  version=20120820
  Output5 : Scope  NumInputPorts=2
  Real-Imag to Complex2 : RealImagToComplex
  Real-Imag to Complex3 : RealImagToComplex
  Smoothing Windpw : DSPBAPrim/DualMem  primtype=dualmem  nInputs=4  nOutputs=2  omode=Inherit via internal rule  otype=sfix(16)  scale=2^-15  rndmethod=Unbiased  factor=1  satmethod=Symmetric  shift_vec=[0 1 2 -1]  value=fi(win,1,16,15)  inPortNames=['d1'; 'a1'; 'w1'; 'a2']  outPortNames=['q1'; 'q2']  dspbaimage=dspba_prim.jpg  text=fprintf('dmem%s',AdvDSPBDMemDisplay(UseDontCare));  style=Optimised  visibilities=8 + 1024 + 2^17  UseDontCare=on  TwinWritePorts=off  version=20141001
  StretchPulse : DSPBAControl/StretchPulse
  StretchPulse1 : DSPBAControl/StretchPulse
  Terminator : Terminator
  Terminator1 : Terminator
  latch_0L : DSPBAControl/latch_0L
  latch_0L1 : DSPBAControl/latch_0L
  cpg_win1 : Outport
  cpg_win2 : Outport  Port=2
  wires:
  Fanout1/2 -> Mult7/1
  Fanout1/1 -> Mult6/1
  Mux1/1 -> Fanout1/1
  Fanout/2 -> Mult3/1
  Fanout/1 -> Mult2/1
  Mux3/1 -> Fanout/1
  LoadableCounter1/1 -> Fanout6/1
  One11/1 -> LoadableCounter1/4
  One12/1 -> LoadableCounter1/3
  One10/1 -> LoadableCounter/4
  One3/1 -> LoadableCounter/3
  Complex to Magnitude-Angle10/1 -> Output5/2
  Data Type Conversion10/1 -> Complex to Magnitude-Angle10/1
  latch_0L/1 -> Mux3/3
  One4/1 -> Mux3/2
  One2/1 -> CmpNE/2
  Convert1/1 -> Mult4/1
  Mult4/1 -> Real-Imag to Complex2/1
  Mult5/1 -> Real-Imag to Complex2/2
  Convert2/1 -> Mult5/1
  Real-Imag to Complex2/1 -> cpg_win1/1, Data Type Conversion10/1
  Smoothing Windpw/1 -> Output5/1, Mult4/2, Mult5/2
  One1/1 -> StretchPulse/2, LoadableCounter/5
  latch_0L1/1 -> Mux1/3
  One9/1 -> Mux1/2
  Smoothing Windpw/2 -> Mult8/2, Mult9/2
  Convert5/1 -> Mult9/1
  Mult6/1 -> Convert3/1
  Convert3/1 -> Mult8/1
  sig_i_d/1 -> Complex to Real-Iag1/1, Complex to Real-Iag3/1
  Mult8/1 -> Real-Imag to Complex3/1
  mag2/1 -> latch_0L1/2, CmpNE1/1
  Mult7/1 -> Convert5/1
  Mult9/1 -> Real-Imag to Complex3/2
  Complex to Real-Iag3/2 -> Mult7/2
  One5/1 -> StretchPulse1/2, LoadableCounter1/5
  One6/1 -> CmpNE1/2
  Complex to Real-Iag3/1 -> Mult6/2
  Complex to Real-Iag1/1 -> Mult2/2
  Mult2/1 -> Convert1/1
  Mult3/1 -> Convert2/1
  Complex to Real-Iag1/2 -> Mult3/2
  Real-Imag to Complex3/1 -> cpg_win2/1
  One7/1 -> Smoothing Windpw/3
  One8/1 -> Smoothing Windpw/1
  mag1/1 -> CmpNE/1, latch_0L/2
  Fanout2/2 -> Mux3/1
  StretchPulse/1 -> Fanout2/1
  Fanout2/1 -> LoadableCounter/1
  Fanout3/2 -> Mux1/1
  StretchPulse1/1 -> Fanout3/1
  Fanout3/1 -> LoadableCounter1/1
  LoadableCounter/1 -> Fanout5/1
  Fanout5/1 -> Smoothing Windpw/2
  Fanout6/1 -> Smoothing Windpw/4
  Fanout5/2 -> Terminator/1
  Fanout6/2 -> Terminator1/1
  CmpNE/1 -> Fanout4/1
  Fanout4/3 -> latch_0L/1
  Fanout4/2 -> StretchPulse/1
  Fanout4/1 -> LoadableCounter/2
  CmpNE1/1 -> Fanout7/1
  Fanout7/3 -> latch_0L1/1
  Fanout7/2 -> StretchPulse1/1
  Fanout7/1 -> LoadableCounter1/2

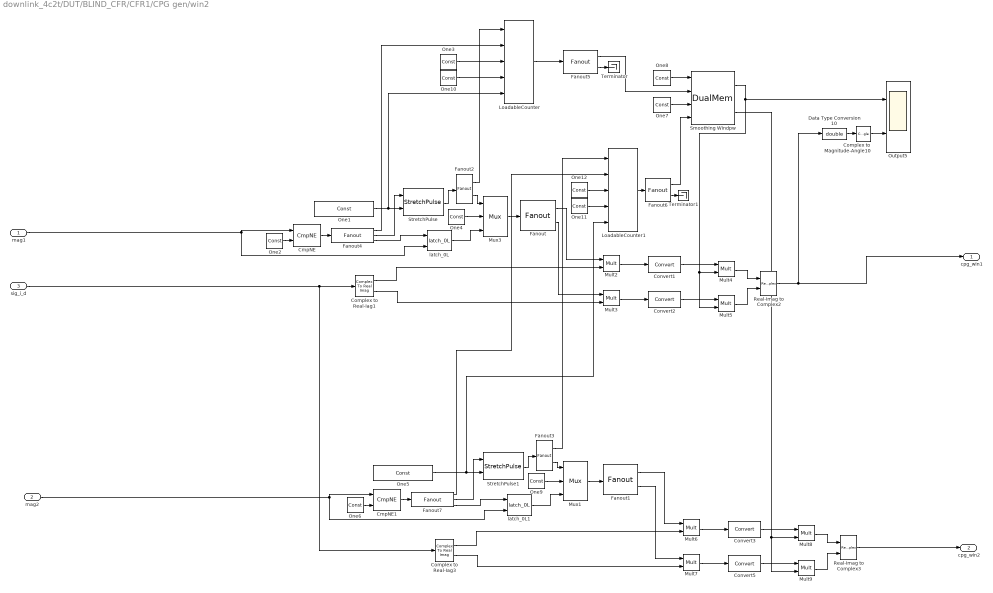
== system downlink_4c2t/DUT/BLIND_CFR/CFR1/CPG gen/win2 ==
  mag1 : Inport
  mag2 : Inport  Port=2
  sig_i_d : Inport  Port=3
  CmpNE : DSPBAPrim/CmpNE  primtype=cmpne  nInputs=2  nOutputs=1  omode=boolean  otype=sfix(16)  scale=2^-15  rndmethod=Unbiased  factor=1  satmethod=Symmetric  shift_vec=[0 1 2 -1]  value=0  inPortNames=[' '; ' ';]  outPortNames=[' ']  dspbaimage=dspba_prim.jpg  text=fprintf('~=');  style=Optimised  visibilities=0  advOptions=[]  version=20130117
  CmpNE1 : DSPBAPrim/CmpNE  primtype=cmpne  nInputs=2  nOutputs=1  omode=boolean  otype=sfix(16)  scale=2^-15  rndmethod=Unbiased  factor=1  satmethod=Symmetric  shift_vec=[0 1 2 -1]  value=0  inPortNames=[' '; ' ';]  outPortNames=[' ']  dspbaimage=dspba_prim.jpg  text=fprintf('~=');  style=Optimised  visibilities=0  advOptions=[]  version=20130117
  Complex to Magnitude-Angle10 : ComplexToMagnitudeAngle  Output=Magnitude
  Complex to Real-Iag1 : ComplexToRealImag
  Complex to Real-Iag3 : ComplexToRealImag
  Convert{1..3,5} (4 alike) : DSPBAPrim/Convert  primtype=convert  nInputs=1  nOutputs=1  omode=Specify via dialog  otype=sfix(16)  scale=2^-(15)  rndmethod=Unbiased  factor=1  satmethod=None  shift_vec=[0 1 2 -1]  value=round([0:255]/17)  inPortNames=[' '; ' ';]  outPortNames=[' '; 'c']  dspbaimage=dspba_prim.jpg  text=fprintf('convert');  style=Optimised  visibilities=8+64+256  clipdetect=off  floatPrecision=float32_m23  advOptions=[]  version=20130211
  Data Type Conversion10 : DataTypeConversion  OutDataTypeStr=double
  Fanout{,1..3,5..6} (6 alike) : DSPBAPrim/Fanout  primtype=fanout  nInputs=1  nOutputs=evalAionMaskParam(gcb,'value',1)  omode=Inherit via internal rule  otype=sfix(16)  scale=2^-15  rndmethod=Unbiased  factor=1  satmethod=Symmetric  shift_vec=[0 1 2 -1]  value=2  inPortNames=[' '; ' ';]  outPortNames=[' ']  dspbaimage=dspba_prim.jpg  text=fprintf('fanout')  style=Optimised  visibilities=2^10+2^18  version=20150501  uninit=off
  Fanout4 : DSPBAPrim/Fanout  primtype=fanout  nInputs=1  nOutputs=evalAionMaskParam(gcb,'value',1)  omode=Inherit via internal rule  otype=sfix(16)  scale=2^-15  rndmethod=Unbiased  factor=1  satmethod=Symmetric  shift_vec=[0 1 2 -1]  value=3  inPortNames=[' '; ' ';]  outPortNames=[' ']  dspbaimage=dspba_prim.jpg  text=fprintf('fanout')  style=Optimised  visibilities=2^10+2^18  version=20150501  uninit=off
  Fanout7 : DSPBAPrim/Fanout  primtype=fanout  nInputs=1  nOutputs=evalAionMaskParam(gcb,'value',1)  omode=Inherit via internal rule  otype=sfix(16)  scale=2^-15  rndmethod=Unbiased  factor=1  satmethod=Symmetric  shift_vec=[0 1 2 -1]  value=3  inPortNames=[' '; ' ';]  outPortNames=[' ']  dspbaimage=dspba_prim.jpg  text=fprintf('fanout')  style=Optimised  visibilities=2^10+2^18  version=20150501  uninit=off
  LoadableCounter : DSPBAPrim/LoadableCounter  primtype=loadablecounter  nInputs=5  nOutputs=1  omode=Inherit via internal rule  otype=ufix(16)  scale=2^-0  rndmethod=Unbiased  factor=1  satmethod=Symmetric  shift_vec=[0 1 2 -1]  value=[0 length(win) 1]  inPortNames=['en';'ld';'i ';'s ';'m ']  outPortNames=[' ']  dspbaimage=dspba_prim.jpg  text=fprintf('loadable\ncounter\n[%d %d %d]', value(1), value(2), value(3));  style=Optimised  visibilities=8 + 1024  version=20090407
  LoadableCounter1 : DSPBAPrim/LoadableCounter  primtype=loadablecounter  nInputs=5  nOutputs=1  omode=Inherit via internal rule  otype=ufix(16)  scale=2^-0  rndmethod=Unbiased  factor=1  satmethod=Symmetric  shift_vec=[0 1 2 -1]  value=[0 length(win) 1]  inPortNames=['en';'ld';'i ';'s ';'m ']  outPortNames=[' ']  dspbaimage=dspba_prim.jpg  text=fprintf('loadable\ncounter\n[%d %d %d]', value(1), value(2), value(3));  style=Optimised  visibilities=8 + 1024  version=20090407
  Mult{2..9} (8 alike) : DSPBAPrim/Mult  primtype=mult  nInputs=2  nOutputs=1  omode=Inherit via internal rule  otype=sfix(16)  scale=2^-15  rndmethod=Unbiased  factor=1  satmethod=Symmetric  shift_vec=[0 1 2 -1]  value=0  inPortNames=[' '; ' ';]  outPortNames=[' ']  dspbaimage=dspba_prim.jpg  text=fprintf('X');  style=Optimised  visibilities=8+2^18+2^19  floatPrecision=float32_m23  floatRounding=correct  advOptions=[]  version=20130115
  Mux1 : DSPBAPrim/Mux  primtype=mux  nInputs=evalAionMaskParam(gcb,'value',1)+1  nOutputs=1  omode=Inherit via internal rule  otype=sfix(16)  scale=2^-15  rndmethod=Unbiased  factor=1  satmethod=Symmetric  shift_vec=[0 1 2 -1]  value=2  inPortNames=['s'; 'd0'; 'd1'; 'd2'; 'd3'; 'd4'; 'd5'; 'd6'; 'd7'; 'd8'; 'd9';]  outPortNames=[' ']  dspbaimage=dspba_prim.jpg  text=fprintf('%s', primtype);  style=Optimised  visibilities=1032  version=20131025
  Mux3 : DSPBAPrim/Mux  primtype=mux  nInputs=evalAionMaskParam(gcb,'value',1)+1  nOutputs=1  omode=Inherit via internal rule  otype=sfix(16)  scale=2^-15  rndmethod=Unbiased  factor=1  satmethod=Symmetric  shift_vec=[0 1 2 -1]  value=2  inPortNames=['s'; 'd0'; 'd1'; 'd2'; 'd3'; 'd4'; 'd5'; 'd6'; 'd7'; 'd8'; 'd9';]  outPortNames=[' ']  dspbaimage=dspba_prim.jpg  text=fprintf('%s', primtype);  style=Optimised  visibilities=1032  version=20131025
  One1 : DSPBAPrim/Const  primtype=const  nInputs=0  nOutputs=1  omode=Specify via dialog  otype=uint(10)  scale=2^0  rndmethod=Unbiased  factor=1  satmethod=Symmetric  shift_vec=[0 1 2 -1]  value=Iter0_Param.winLen  inPortNames=['+'; '+';]  outPortNames=[' ']  dspbaimage=dspba_prim.jpg  text=fprintf('%s', num2str(value));  style=Optimised  visibilities=8 + 1024  floatPrecision=float32_m23  version=20120820
  One10 : DSPBAPrim/Const  primtype=const  nInputs=0  nOutputs=1  omode=Specify via dialog  otype=uint(10)  scale=2^0  rndmethod=Unbiased  factor=1  satmethod=Symmetric  shift_vec=[0 1 2 -1]  value=1  inPortNames=['+'; '+';]  outPortNames=[' ']  dspbaimage=dspba_prim.jpg  text=fprintf('%s', num2str(value));  style=Optimised  visibilities=8 + 1024  floatPrecision=float32_m23  version=20120820
  One11 : DSPBAPrim/Const  primtype=const  nInputs=0  nOutputs=1  omode=Specify via dialog  otype=uint(10)  scale=2^0  rndmethod=Unbiased  factor=1  satmethod=Symmetric  shift_vec=[0 1 2 -1]  value=1  inPortNames=['+'; '+';]  outPortNames=[' ']  dspbaimage=dspba_prim.jpg  text=fprintf('%s', num2str(value));  style=Optimised  visibilities=8 + 1024  floatPrecision=float32_m23  version=20120820
  One12 : DSPBAPrim/Const  primtype=const  nInputs=0  nOutputs=1  omode=Specify via dialog  otype=uint(10)  scale=2^0  rndmethod=Unbiased  factor=1  satmethod=Symmetric  shift_vec=[0 1 2 -1]  value=0  inPortNames=['+'; '+';]  outPortNames=[' ']  dspbaimage=dspba_prim.jpg  text=fprintf('%s', num2str(value));  style=Optimised  visibilities=8 + 1024  floatPrecision=float32_m23  version=20120820
  One2 : DSPBAPrim/Const  primtype=const  nInputs=0  nOutputs=1  omode=Inherit via internal rule  otype=sfix(16)  scale=2^-15  rndmethod=Unbiased  factor=1  satmethod=Symmetric  shift_vec=[0 1 2 -1]  value=0  inPortNames=['+'; '+';]  outPortNames=[' ']  dspbaimage=dspba_prim.jpg  text=fprintf('%s', num2str(value));  style=Optimised  visibilities=8 + 1024  floatPrecision=float32_m23  version=20120820
  One3 : DSPBAPrim/Const  primtype=const  nInputs=0  nOutputs=1  omode=Specify via dialog  otype=uint(10)  scale=2^0  rndmethod=Unbiased  factor=1  satmethod=Symmetric  shift_vec=[0 1 2 -1]  value=0  inPortNames=['+'; '+';]  outPortNames=[' ']  dspbaimage=dspba_prim.jpg  text=fprintf('%s', num2str(value));  style=Optimised  visibilities=8 + 1024  floatPrecision=float32_m23  version=20120820
  One4 : DSPBAPrim/Const  primtype=const  nInputs=0  nOutputs=1  omode=Specify via dialog  otype=ufix(16)  scale=2^-15  rndmethod=Unbiased  factor=1  satmethod=Symmetric  shift_vec=[0 1 2 -1]  value=0  inPortNames=['+'; '+';]  outPortNames=[' ']  dspbaimage=dspba_prim.jpg  text=fprintf('%s', num2str(value));  style=Optimised  visibilities=8 + 1024  floatPrecision=float32_m23  version=20120820
  One5 : DSPBAPrim/Const  primtype=const  nInputs=0  nOutputs=1  omode=Specify via dialog  otype=uint(10)  scale=2^0  rndmethod=Unbiased  factor=1  satmethod=Symmetric  shift_vec=[0 1 2 -1]  value=Iter0_Param.winLen  inPortNames=['+'; '+';]  outPortNames=[' ']  dspbaimage=dspba_prim.jpg  text=fprintf('%s', num2str(value));  style=Optimised  visibilities=8 + 1024  floatPrecision=float32_m23  version=20120820
  One6 : DSPBAPrim/Const  primtype=const  nInputs=0  nOutputs=1  omode=Inherit via internal rule  otype=sfix(16)  scale=2^-15  rndmethod=Unbiased  factor=1  satmethod=Symmetric  shift_vec=[0 1 2 -1]  value=0  inPortNames=['+'; '+';]  outPortNames=[' ']  dspbaimage=dspba_prim.jpg  text=fprintf('%s', num2str(value));  style=Optimised  visibilities=8 + 1024  floatPrecision=float32_m23  version=20120820
  One7 : DSPBAPrim/Const  primtype=const  nInputs=0  nOutputs=1  omode=boolean  otype=sfix(16)  scale=2^-15  rndmethod=Unbiased  factor=1  satmethod=Symmetric  shift_vec=[0 1 2 -1]  value=0  inPortNames=['+'; '+';]  outPortNames=[' ']  dspbaimage=dspba_prim.jpg  text=fprintf('%s', num2str(value));  style=Optimised  visibilities=8 + 1024  floatPrecision=float32_m23  version=20120820
  One8 : DSPBAPrim/Const  primtype=const  nInputs=0  nOutputs=1  omode=Specify via dialog  otype=sfix(16)  scale=2^-15  rndmethod=Unbiased  factor=1  satmethod=Symmetric  shift_vec=[0 1 2 -1]  value=0  inPortNames=['+'; '+';]  outPortNames=[' ']  dspbaimage=dspba_prim.jpg  text=fprintf('%s', num2str(value));  style=Optimised  visibilities=8 + 1024  floatPrecision=float32_m23  version=20120820
  One9 : DSPBAPrim/Const  primtype=const  nInputs=0  nOutputs=1  omode=Specify via dialog  otype=ufix(16)  scale=2^-15  rndmethod=Unbiased  factor=1  satmethod=Symmetric  shift_vec=[0 1 2 -1]  value=0  inPortNames=['+'; '+';]  outPortNames=[' ']  dspbaimage=dspba_prim.jpg  text=fprintf('%s', num2str(value));  style=Optimised  visibilities=8 + 1024  floatPrecision=float32_m23  version=20120820
  Output5 : Scope  NumInputPorts=2
  Real-Imag to Complex2 : RealImagToComplex
  Real-Imag to Complex3 : RealImagToComplex
  Smoothing Windpw : DSPBAPrim/DualMem  primtype=dualmem  nInputs=4  nOutputs=2  omode=Inherit via internal rule  otype=sfix(16)  scale=2^-15  rndmethod=Unbiased  factor=1  satmethod=Symmetric  shift_vec=[0 1 2 -1]  value=fi(win,1,16,15)  inPortNames=['d1'; 'a1'; 'w1'; 'a2']  outPortNames=['q1'; 'q2']  dspbaimage=dspba_prim.jpg  text=fprintf('dmem%s',AdvDSPBDMemDisplay(UseDontCare));  style=Optimised  visibilities=8 + 1024 + 2^17  UseDontCare=on  TwinWritePorts=off  version=20141001
  StretchPulse : DSPBAControl/StretchPulse
  StretchPulse1 : DSPBAControl/StretchPulse
  Terminator : Terminator
  Terminator1 : Terminator
  latch_0L : DSPBAControl/latch_0L
  latch_0L1 : DSPBAControl/latch_0L
  cpg_win1 : Outport
  cpg_win2 : Outport  Port=2
  wires:
  Fanout7/1 -> LoadableCounter1/2
  Fanout7/2 -> StretchPulse1/1
  Fanout7/3 -> latch_0L1/1
  CmpNE1/1 -> Fanout7/1
  Fanout4/1 -> LoadableCounter/2
  Fanout4/2 -> StretchPulse/1
  Fanout4/3 -> latch_0L/1
  CmpNE/1 -> Fanout4/1
  Fanout6/2 -> Terminator1/1
  Fanout5/2 -> Terminator/1
  Fanout6/1 -> Smoothing Windpw/4
  Fanout5/1 -> Smoothing Windpw/2
  LoadableCounter/1 -> Fanout5/1
  Fanout3/1 -> LoadableCounter1/1
  StretchPulse1/1 -> Fanout3/1
  Fanout3/2 -> Mux1/1
  Fanout2/1 -> LoadableCounter/1
  StretchPulse/1 -> Fanout2/1
  Fanout2/2 -> Mux3/1
  mag1/1 -> latch_0L/2, CmpNE/1
  One8/1 -> Smoothing Windpw/1
  One7/1 -> Smoothing Windpw/3
  Real-Imag to Complex3/1 -> cpg_win2/1
  Complex to Real-Iag1/2 -> Mult3/2
  Mult3/1 -> Convert2/1
  Mult2/1 -> Convert1/1
  Complex to Real-Iag1/1 -> Mult2/2
  Complex to Real-Iag3/1 -> Mult6/2
  One6/1 -> CmpNE1/2
  One5/1 -> LoadableCounter1/5, StretchPulse1/2
  Complex to Real-Iag3/2 -> Mult7/2
  Mult9/1 -> Real-Imag to Complex3/2
  Mult7/1 -> Convert5/1
  mag2/1 -> CmpNE1/1, latch_0L1/2
  Mult8/1 -> Real-Imag to Complex3/1
  sig_i_d/1 -> Complex to Real-Iag3/1, Complex to Real-Iag1/1
  Convert3/1 -> Mult8/1
  Mult6/1 -> Convert3/1
  Convert5/1 -> Mult9/1
  Smoothing Windpw/2 -> Mult9/2, Mult8/2
  One9/1 -> Mux1/2
  latch_0L1/1 -> Mux1/3
  One1/1 -> LoadableCounter/5, StretchPulse/2
  Smoothing Windpw/1 -> Mult5/2, Mult4/2, Output5/1
  Real-Imag to Complex2/1 -> Data Type Conversion10/1, cpg_win1/1
  Convert2/1 -> Mult5/1
  Mult5/1 -> Real-Imag to Complex2/2
  Mult4/1 -> Real-Imag to Complex2/1
  Convert1/1 -> Mult4/1
  One2/1 -> CmpNE/2
  One4/1 -> Mux3/2
  latch_0L/1 -> Mux3/3
  Data Type Conversion10/1 -> Complex to Magnitude-Angle10/1
  Complex to Magnitude-Angle10/1 -> Output5/2
  One3/1 -> LoadableCounter/3
  One10/1 -> LoadableCounter/4
  One12/1 -> LoadableCounter1/3
  One11/1 -> LoadableCounter1/4
  LoadableCounter1/1 -> Fanout6/1
  Mux3/1 -> Fanout/1
  Fanout/1 -> Mult2/1
  Fanout/2 -> Mult3/1
  Mux1/1 -> Fanout1/1
  Fanout1/1 -> Mult6/1
  Fanout1/2 -> Mult7/1
